simulink model "Antons_Attempt"  (R2023b)
settings: Solver=VariableStepAuto  StartTime=0.0  StopTime=1.0  RelTol=1e-3
settings Model: Creator=FIRSTMentor  LastModifiedBy=FIRSTMentor

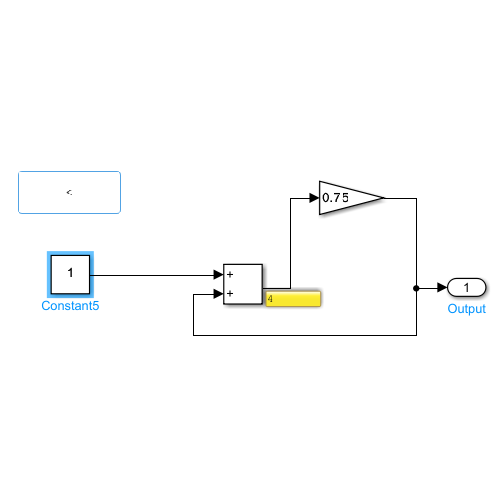
[thumbnail: Simulink's stored preview of the top-level diagram]
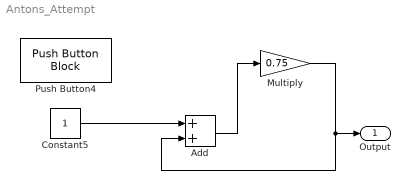
== system Antons_Attempt ==
  Add : Sum
  Constant5 : Constant
  Multiply : Gain  Gain=0.75
  Push Button4 : PushButtonBlock  ButtonText=<  OffValue=0.000000
  Output : Outport
  wires:
  Constant5/1 -> Add/1
  Multiply/1 -> Output/1, Add/2
  Add/1 -> Multiply/1
